simulink model "Lab1"  (R2023b)
settings: Solver=VariableStepAuto  StartTime=0.0  StopTime=10.0  RelTol=1e-3
settings Model: Creator=gaafa  LastModifiedBy=gaafa

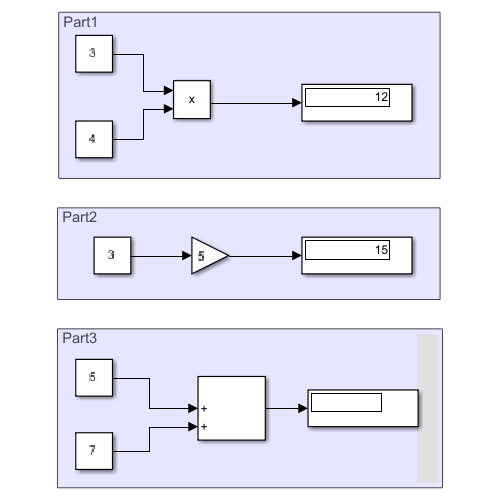
[thumbnail: Simulink's stored preview of the top-level diagram]
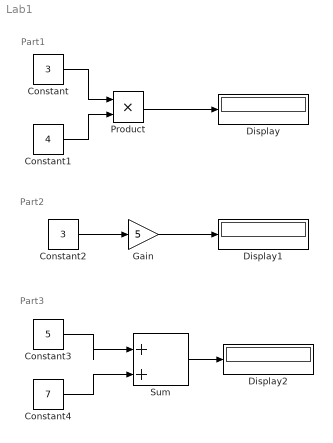
== system Lab1 ==
  note: Part3
  note: Part2
  note: Part1
  Constant : Constant  Value=3
  Constant1 : Constant  Value=4
  Constant2 : Constant  Value=3
  Constant3 : Constant  Value=5
  Constant4 : Constant  Value=7
  Display : Display
  Display1 : Display
  Display2 : Display
  Gain : Gain  Gain=5
  Product : Product
  Sum : Sum  Inputs=|++
  wires:
  Constant/1 -> Product/1
  Constant1/1 -> Product/2
  Product/1 -> Display/1
  Constant2/1 -> Gain/1
  Gain/1 -> Display1/1
  Constant3/1 -> Sum/1
  Constant4/1 -> Sum/2
  Sum/1 -> Display2/1
